simulink model "schema_di_controlloC1_Pelliccia_Tornabene_Valmaggi"  (R2023b)
settings: Solver=VariableStepAuto  StartTime=0.0  StopTime=0.02  RelTol=1e-3
values from neighbouring files (symbols this model uses):
  C = [1 0]    [CAT_ProgettoC1_Tornabene_Valmaggi_Pelliccia.m]
  DD = 1    [CAT_ProgettoC1_Tornabene_Valmaggi_Pelliccia.m]
  kk = 1:4    [CAT_ProgettoC1_Tornabene_Valmaggi_Pelliccia.m]
  NN = 0.2    [CAT_ProgettoC1_Tornabene_Valmaggi_Pelliccia.m]
  omega_d = 0.01    [CAT_ProgettoC1_Tornabene_Valmaggi_Pelliccia.m]
  omega_n = omega_n_min    (= 80000)    [CAT_ProgettoC1_Tornabene_Valmaggi_Pelliccia.m]
  u_e = m*9.81 + k*x1_e    (= 199525)    [CAT_ProgettoC1_Tornabene_Valmaggi_Pelliccia.m]
  x1_e = 0.35    [CAT_ProgettoC1_Tornabene_Valmaggi_Pelliccia.m]
  x2_e = 0    [CAT_ProgettoC1_Tornabene_Valmaggi_Pelliccia.m]
libraries: cstblocks x2
settings Model: Creator=enrico  LastModifiedBy=enrico

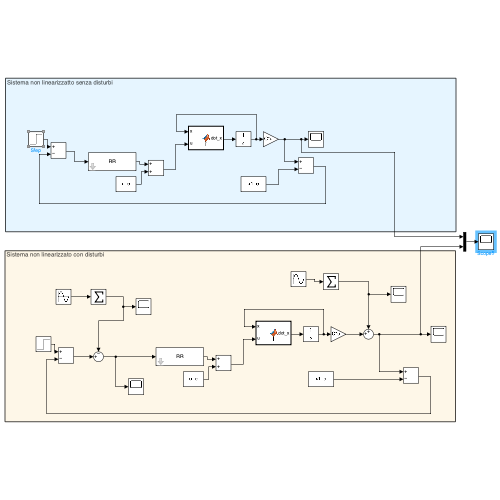
[thumbnail: Simulink's stored preview of the top-level diagram]
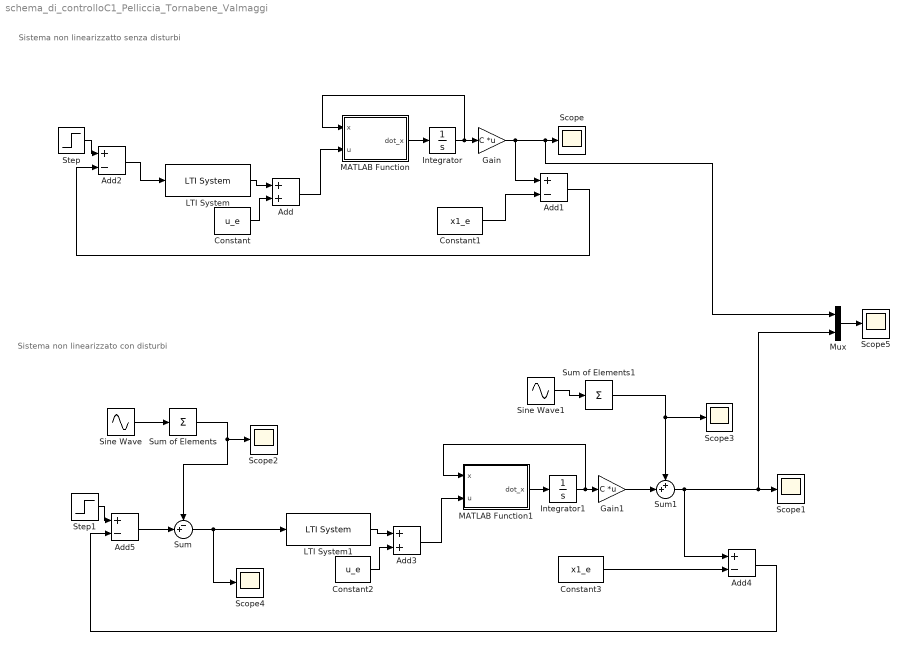
== system schema_di_controlloC1_Pelliccia_Tornabene_Valmaggi ==
  note: Sistema non linearizzato con disturbi
  note: Sistema non linearizzatto senza disturbi
  Add : Sum
  Add{1..2,4..5} (4 alike) : Sum  Inputs=+-
  Add3 : Sum
  Constant : Constant  Value=u_e
  Constant1 : Constant  Value=x1_e
  Constant2 : Constant  Value=u_e
  Constant3 : Constant  Value=x1_e
  Gain : Gain  Gain=C  Multiplication=Matrix(K*u)
  Gain1 : Gain  Gain=C  Multiplication=Matrix(K*u)
  Integrator : Integrator  InitialCondition=[x1_e; x2_e]
  Integrator1 : Integrator  InitialCondition=[x1_e; x2_e]
  LTI System : cstblocks/LTI System  sys=RR  IC=[]  PadeOrder=0
  LTI System1 : cstblocks/LTI System  sys=RR  IC=[]  PadeOrder=0
  MATLAB Function : MATLAB Function  TreatAsAtomicUnit=on
  MATLAB Function1 : MATLAB Function  TreatAsAtomicUnit=on
  Mux : Mux  Inputs=2
  Scope{,1..5} (6 alike) : Scope
  Sine Wave : Sin  Amplitude=NN  Frequency=omega_n*kk  SampleTime=0
  Sine Wave1 : Sin  Amplitude=DD  Frequency=omega_d*kk  SampleTime=0
  Step : Step  Time=0  SampleTime=0
  Step1 : Step  Time=0  SampleTime=0
  Sum : Sum  Inputs=-+|
  Sum of Elements : Sum  Inputs=+
  Sum of Elements1 : Sum  Inputs=+  CollapseDim=4
  Sum1 : Sum  Inputs=++|
  wires:
  Add1/1 -> Add2/2
  Add/1 -> MATLAB Function/2(u)
  LTI System/1 -> Add/1
  Step/1 -> Add2/1
  Add2/1 -> LTI System/1
  Constant1/1 -> Add1/2
  MATLAB Function/1(dot_x) -> Integrator/1
  Gain/1 -> Add1/1, Mux/1, Scope/1
  Integrator/1 -> MATLAB Function/1(x), Gain/1
  Constant/1 -> Add/2
  Integrator1/1 -> MATLAB Function1/1(x), Gain1/1
  LTI System1/1 -> Add3/1
  Constant3/1 -> Add4/2
  MATLAB Function1/1(dot_x) -> Integrator1/1
  Add3/1 -> MATLAB Function1/2(u)
  Add4/1 -> Add5/2
  Step1/1 -> Add5/1
  Add5/1 -> Sum/2
  Constant2/1 -> Add3/2
  Sum/1 -> Scope4/1, LTI System1/1
  Sine Wave/1 -> Sum of Elements/1
  Sum of Elements/1 -> Sum/1, Scope2/1
  Sum of Elements1/1 -> Scope3/1, Sum1/1
  Gain1/1 -> Sum1/2
  Sum1/1 -> Mux/2, Scope1/1, Add4/1
  Sine Wave1/1 -> Sum of Elements1/1
  Mux/1 -> Scope5/1

== matlab function schema_di_controlloC1_Pelliccia_Tornabene_Valmaggi/MATLAB Function ==
  data: x input; u input; dot_x output
function dot_x = f(x,u)

m = 2500;   % Massa
beta = 0.1; % Coefficiente di non linearità della molla
n = 3;      % Coefficiente di non linearità della molla
k = 5 * 1e5;% Costante elastica lineare della molla
b = 350;    % Coefficiente di attrito dinamico
g = 9.81;   % Acc. gravitazionale

dot_x = zeros(2,1);
dot_x(1) = x(2);
dot_x(2) = - g - (b/m) * x(2) - (k/m) * x(1) - (beta/m) * (x(2)^3 + n * x(2) * sin(n*x(2))^2 ) + (u / m);

== matlab function schema_di_controlloC1_Pelliccia_Tornabene_Valmaggi/MATLAB Function1 ==
  data: x input; u input; dot_x output
function dot_x = f(x,u)

m = 2500;   % Massa
beta = 0.1; % Coefficiente di non linearità della molla
n = 3;      % Coefficiente di non linearità della molla
k = 5 * 1e5;% Costante elastica lineare della molla
b = 350;    % Coefficiente di attrito dinamico
g = 9.81;   % Acc. gravitazionale

dot_x = zeros(2,1);
dot_x(1) = x(2);
dot_x(2) = - g - (b/m) * x(2) - (k/m) * x(1) - (beta/m) * (x(2)^3 + n * x(2) * sin(n*x(2))^2 ) + (u / m);
